simulink library "ammclib_bam_S32K11x"  (R2016a)
settings: Solver=VariableStepAuto  SolverMode=SingleTasking  StartTime=0.0  StopTime=10.0  RelTol=1e-3
undefined symbols (not defined in the file or in its folder): f16A1, f16A2, f16ADCMaxError, f16B0, f16B1, f16B2, f16C1, f16CC1, f16CC1sc, f16CC1sc_D, f16CC1sc_Q, f16CC2, f16CC2sc, f16CC2sc_D, f16CC2sc_Q, f16DerivGain, f16EGain, f16FiltCoef, f16HystOff, f16HystOn, f16IGain, f16IntegGain, f16IntegGainFW, f16IntegGainQ, f16Kd, f16Kq, f16Limit, f16LowerLimit, f16LowerLimit_D, f16LowerLimit_Q, f16LowerLimitFW, f16LowerLimitQ, f16ModIndex, f16OutValOff, f16OutValOn, f16PropGain, f16PropGainFW, f16PropGainQ, f16RampDown, f16RampUp, f16UGain, f16UpperLimit, f16UpperLimit_D, f16UpperLimit_Q, f16UpperLimitFW, f16UpperLimitQ, f16WIGain, f32A1, f32A2, f32ADCMaxError, f32B0, f32B1, f32B2, f32C1, f32CC1, f32CC1sc, f32CC1sc_D, f32CC1sc_Q, f32CC2, f32CC2sc ... (+62)
(part 16 of 16)

== system ammclib_bam_S32K11x/MLIB/F32/MLIB_MacSat_F32/copyright ==

== system ammclib_bam_S32K11x/MLIB/F32/MLIB_MacSat_F32/copyright2 ==

== system ammclib_bam_S32K11x/MLIB/F32/MLIB_Mac_F32/copyright ==

== system ammclib_bam_S32K11x/MLIB/F32/MLIB_Mac_F32/copyright2 ==

== system ammclib_bam_S32K11x/MLIB/F32/MLIB_Mnac_F32/copyright ==

== system ammclib_bam_S32K11x/MLIB/F32/MLIB_Mnac_F32/copyright2 ==

== system ammclib_bam_S32K11x/MLIB/F32/MLIB_Msu_F32/copyright ==

== system ammclib_bam_S32K11x/MLIB/F32/MLIB_Msu_F32/copyright2 ==

== system ammclib_bam_S32K11x/MLIB/F32/MLIB_MulSat_F32/copyright ==

== system ammclib_bam_S32K11x/MLIB/F32/MLIB_MulSat_F32/copyright2 ==

== system ammclib_bam_S32K11x/MLIB/F32/MLIB_Mul_F32/copyright ==

== system ammclib_bam_S32K11x/MLIB/F32/MLIB_Mul_F32/copyright2 ==

== system ammclib_bam_S32K11x/MLIB/F32/MLIB_NegSat_F32/copyright ==

== system ammclib_bam_S32K11x/MLIB/F32/MLIB_NegSat_F32/copyright2 ==

== system ammclib_bam_S32K11x/MLIB/F32/MLIB_Neg_F32/copyright ==

== system ammclib_bam_S32K11x/MLIB/F32/MLIB_Neg_F32/copyright2 ==

== system ammclib_bam_S32K11x/MLIB/F32/MLIB_Norm_F32/copyright ==

== system ammclib_bam_S32K11x/MLIB/F32/MLIB_Norm_F32/copyright2 ==

== system ammclib_bam_S32K11x/MLIB/F32/MLIB_Round_F32/copyright ==

== system ammclib_bam_S32K11x/MLIB/F32/MLIB_Round_F32/copyright2 ==

== system ammclib_bam_S32K11x/MLIB/F32/MLIB_ShBiSat_F32/copyright ==

== system ammclib_bam_S32K11x/MLIB/F32/MLIB_ShBiSat_F32/copyright2 ==

== system ammclib_bam_S32K11x/MLIB/F32/MLIB_ShBi_F32/copyright ==

== system ammclib_bam_S32K11x/MLIB/F32/MLIB_ShBi_F32/copyright2 ==

== system ammclib_bam_S32K11x/MLIB/F32/MLIB_ShLSat_F32/copyright ==

== system ammclib_bam_S32K11x/MLIB/F32/MLIB_ShLSat_F32/copyright2 ==

== system ammclib_bam_S32K11x/MLIB/F32/MLIB_ShL_F32/copyright ==

== system ammclib_bam_S32K11x/MLIB/F32/MLIB_ShL_F32/copyright2 ==

== system ammclib_bam_S32K11x/MLIB/F32/MLIB_ShR_F32/copyright ==

== system ammclib_bam_S32K11x/MLIB/F32/MLIB_ShR_F32/copyright2 ==

== system ammclib_bam_S32K11x/MLIB/F32/MLIB_SubSat_F32/copyright ==

== system ammclib_bam_S32K11x/MLIB/F32/MLIB_SubSat_F32/copyright2 ==

== system ammclib_bam_S32K11x/MLIB/F32/MLIB_Sub_F32/copyright ==

== system ammclib_bam_S32K11x/MLIB/F32/MLIB_Sub_F32/copyright2 ==

== system ammclib_bam_S32K11x/MLIB/F32/MLIB_VAdd_F32/copyright ==

== system ammclib_bam_S32K11x/MLIB/F32/MLIB_VAdd_F32/copyright2 ==

== system ammclib_bam_S32K11x/MLIB/F32/MLIB_VMac_F32/copyright ==

== system ammclib_bam_S32K11x/MLIB/F32/MLIB_VMac_F32/copyright2 ==

== system ammclib_bam_S32K11x/MLIB/F32/MLIB_VScale_F32/copyright ==

== system ammclib_bam_S32K11x/MLIB/F32/MLIB_VScale_F32/copyright2 ==

== system ammclib_bam_S32K11x/MLIB/F32/MLIB_VSub_F32/copyright ==

== system ammclib_bam_S32K11x/MLIB/F32/MLIB_VSub_F32/copyright2 ==

== system ammclib_bam_S32K11x/MLIB/F32F16F16/MLIB_MacSat_F32F16F16/copyright ==

== system ammclib_bam_S32K11x/MLIB/F32F16F16/MLIB_MacSat_F32F16F16/copyright2 ==

== system ammclib_bam_S32K11x/MLIB/F32F16F16/MLIB_Mac_F32F16F16/copyright ==

== system ammclib_bam_S32K11x/MLIB/F32F16F16/MLIB_Mac_F32F16F16/copyright2 ==

== system ammclib_bam_S32K11x/MLIB/F32F16F16/MLIB_Mnac_F32F16F16/copyright ==

== system ammclib_bam_S32K11x/MLIB/F32F16F16/MLIB_Mnac_F32F16F16/copyright2 ==

== system ammclib_bam_S32K11x/MLIB/F32F16F16/MLIB_Msu_F32F16F16/copyright ==

== system ammclib_bam_S32K11x/MLIB/F32F16F16/MLIB_Msu_F32F16F16/copyright2 ==

== system ammclib_bam_S32K11x/MLIB/F32F16F16/MLIB_MulSat_F32F16F16/copyright ==

== system ammclib_bam_S32K11x/MLIB/F32F16F16/MLIB_MulSat_F32F16F16/copyright2 ==

== system ammclib_bam_S32K11x/MLIB/F32F16F16/MLIB_Mul_F32F16F16/copyright ==

== system ammclib_bam_S32K11x/MLIB/F32F16F16/MLIB_Mul_F32F16F16/copyright2 ==

== system ammclib_bam_S32K11x/MLIB/F32F16F16/MLIB_VMac_F32F16F16/copyright ==

== system ammclib_bam_S32K11x/MLIB/F32F16F16/MLIB_VMac_F32F16F16/copyright2 ==
